simulink model "serial_leg_6dof_demo"  (R2024b)
settings: Solver=ode4  StartTime=0.0  StopTime=4  FixedStep=0.001  RelTol=1e-3
model workspace (MAT data in the model file):
  A6 = [0  1  0  0  0  0; 479.811080876  0  0  0  6.2873101462  0; 0  0  0  1  0  0; -129.668427915  0  0  0  -0.356280908285  0; 0  0  0  0  0  1; 33.3482328696  0  0  0  26.4472963583  0]
  B6 = [0  0; -57.2680605582  11.1276705166; 0  0; 16.5785234316  -2.85279021816; 0  0; -1.40611359443  3.76501844685]
  C6 = [1  0  0  0  0  0; 0  1  0  0  0  0; 0  0  1  0  0  0; 0  0  0  1  0  0; 0  0  0  0  1  0; 0  0  0  0  0  1]
  D6 = [0  0; 0  0; 0  0; 0  0; 0  0; 0  0]
  K6 = [-20.137234893  -2.57738700323  -0.165954300096  -3.79426606162  12.1086875076  1.83005716914; 52.53043904  8.19707414043  0.670211463342  15.2765009018  39.9546309954  2.23927503471]
  x0 = [0; 0; 0; 0; 0.174532925199; 0]
settings Model: Creator=LENOVO  LastModifiedBy=LENOVO

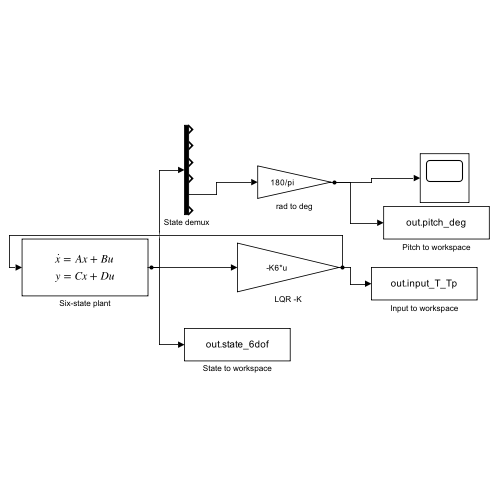
[thumbnail: Simulink's stored preview of the top-level diagram]
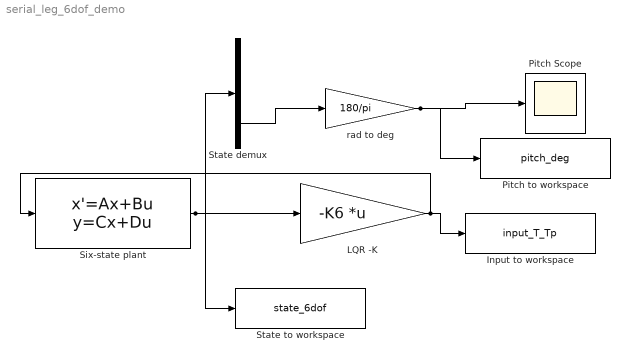
== system serial_leg_6dof_demo ==
  Input to workspace : ToWorkspace  VariableName=input_T_Tp  SaveFormat=Timeseries  SampleTime=-1
  LQR -K : Gain  Gain=-K6  Multiplication=Matrix(K*u)
  Pitch Scope : Scope
  Pitch to workspace : ToWorkspace  VariableName=pitch_deg  SaveFormat=Timeseries  SampleTime=-1
  Six-state plant : StateSpace  A=A6  B=B6  C=C6  D=D6  InitialCondition=x0
  State demux : Demux  Outputs=6
  State to workspace : ToWorkspace  VariableName=state_6dof  SaveFormat=Timeseries  SampleTime=-1
  rad to deg : Gain  Gain=180/pi
  wires:
  Six-state plant/1 -> LQR -K/1, State demux/1, State to workspace/1
  LQR -K/1 -> Six-state plant/1, Input to workspace/1
  State demux/5 -> rad to deg/1
  rad to deg/1 -> Pitch Scope/1, Pitch to workspace/1
